simulink model "gm_parallel_lht"  (R2019b)
settings: Solver=FixedStepDiscrete  StartTime=0.0  StopTime=inf  RelTol=1e-3
undefined symbols (not defined in the file or in its folder): bt, height, width
libraries: hdlsllib x190, simulink x13, hdlmdlgenlib x7, dspsrcs4 x1
(part 18 of 18)

== matlab function gm_parallel_lht/Parallel LHT/Parallel LHT Accumulator/Accumulator Controller/Accumulator Controller ==
  data: sof input; mode output; eof input; read output; clear output; index output; ntheta input; nrho input; valid output
function [mode, read, clear, index, valid] = fcn(sof, eof, ntheta, nrho)

IDLE = fi(0, 0, 2, 0);
VOTE = fi(1, 0, 2, 0);
READ = fi(2, 0, 2, 0);
CLEAR = fi(3, 0, 2, 0);

persistent current_state;
persistent rho_counter;
persistent theta_counter;

if isempty(current_state)
    current_state = IDLE;
end

if isempty(rho_counter)
    rho_counter = fi(0, 0, 16, 0);
end

if isempty(theta_counter)
    theta_counter = fi(0, 0, 16, 0);
end

switch current_state
    case IDLE
        rho_counter = fi(0, 0, 16, 0);
        theta_counter = fi(0, 0, 16, 0);
        
        clear = false;
        read = rho_counter;
        index = theta_counter;
        valid = false;
        
        if sof
            mode = true;
            current_state = VOTE;
        else
            mode = false;
            current_state = IDLE;
        end
        
    case VOTE
        rho_counter = fi(0, 0, 16, 0);
        theta_counter = fi(0, 0, 16, 0);
        
        mode = true;
        clear = false;
        valid = false;
        
        read = rho_counter;
        index = theta_counter;
        
        if eof
            current_state = READ;
        else
            current_state = VOTE;
        end
        
    case READ
        mode = false;
        clear = false;
        read = rho_counter;
        index = theta_counter;
        valid = true;
        
        if theta_counter >= nrho && rho_counter >= ntheta
            rho_counter = fi(0, 0, 16, 0);
            theta_counter = fi(0, 0, 16, 0);
            current_state = CLEAR;
        elseif rho_counter >= nrho
            theta_counter = fi(theta_counter + 1, 0, 16, 0);
            rho_counter = fi(0, 0, 16, 0);
            current_state = READ;
        else
            rho_counter = fi(rho_counter + 1, 0, 16, 0);
            current_state = READ;
        end
        
    case CLEAR
        mode = false;
        clear = true;
        valid = false;
        
        read = rho_counter;
        index = theta_counter;
        
        if rho_counter >= nrho
            rho_counter = fi(0, 0, 16, 0);
            theta_counter = fi(0, 0, 16, 0);
            current_state = IDLE;
        else
            rho_counter = fi(rho_counter + 1, 0, 16, 0);
            theta_counter = fi(0, 0, 16, 0);
            current_state = CLEAR;
        end
        
    otherwise
        rho_counter = fi(0, 0, 16, 0);
        theta_counter = fi(0, 0, 16, 0);
        
        mode = false;
        clear = false;
        valid = false;
        
        read = rho_counter;
        index = theta_counter;
        
        current_state = IDLE;
        
end

== matlab function gm_parallel_lht/Parallel LHT/Parallel LHT Kernel/Hough Kernel/Hough Kernel Symmetric Look Ahead/Look Ahead Hough/MATLAB Function/MATLAB Function ==
  data: index output; eol input; sel output; write output; ntheta input; debug_state output
function [index, sel, write, debug_state] = fcn(eol, ntheta)

BANK = fi(1, 0, 3, 0);
WAIT = fi(2, 0, 3, 0);

persistent state;

persistent thetacounter;

if isempty(state)
    state = BANK;
end

if isempty(thetacounter)
    thetacounter = fi(0, 0, 16, 0);
end

switch state
    case BANK
        sel = false;
        write = true;
        index = thetacounter;
        debug_state = state;
        
        if thetacounter == ntheta
            thetacounter = fi(0, 0, 16, 0);
            state = WAIT;
        else
            thetacounter = fi(thetacounter + 1, 0, 16, 0);
            state = BANK;
        end
        
    case WAIT
        write = false;
        index = thetacounter;
        debug_state = state;
        
        thetacounter = fi(0, 0, 16, 0);
        
        if eol
            sel = true;
            state = BANK;
        else
            sel = false;
            state = WAIT;
        end
        
    otherwise
        thetacounter = fi(0, 0, 16, 0);
        sel = false;
        write = false;
        index = thetacounter;
        debug_state = state;
        
        state = WAIT;
        
end
